simulink model "time_headway"  (R2019b)
settings: Solver=VariableStepAuto  StartTime=0.0  StopTime=10.0  RelTol=1e-3
libraries: robotlib x4
settings Model: Creator=ivory  LastModifiedBy=ivory

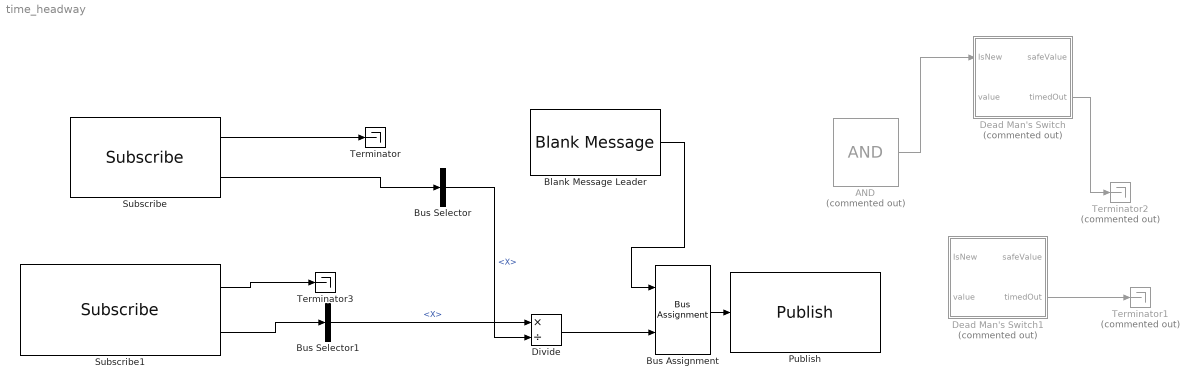
== system time_headway ==
  AND : Logic  Commented=on  IconShape=distinctive  AllPortsSameDT=off  OutDataTypeStr=boolean
  Blank Message Leader : robotlib/Blank Message  messageClass=Message  entityType=std_msgs/Float64  messageType=std_msgs/Float64  SampleTime=inf
      settings: SourceProductName=ROS Toolbox
  Bus Assignment : BusAssignment  AssignedSignals=Data
  Bus Selector : BusSelector  OutputSignals=Twist.Linear.X
  Bus Selector1 : BusSelector  OutputSignals=Point.X
  Dead Man's Switch : Subsystem  Commented=on  TreatAsAtomicUnit=on  mask{stepSize=0.05, timeout=0.2}
      mask prompts: stepSize "Simulation step size"; timeout "Timeout (in seconds)"
      mask help: Interprets whether a new message has been recently received, and if so permits the data in 'value' to be passed through. Otherwise, 0 is outputted from 'safeValue'
      mask Help: Interprets whether a new message has been recently received, and if so permits the data in 'value' to be passed through. Otherwise, 0 is outputted from 'safeValue'
  Dead Man's Switch1 : Subsystem  Commented=on  TreatAsAtomicUnit=on  mask{stepSize=0.05, timeout=0.2}
      mask prompts: stepSize "Simulation step size"; timeout "Timeout (in seconds)"
      mask help: Interprets whether a new message has been recently received, and if so permits the data in 'value' to be passed through. Otherwise, 0 is outputted from 'safeValue'
      mask Help: Interprets whether a new message has been recently received, and if so permits the data in 'value' to be passed through. Otherwise, 0 is outputted from 'safeValue'
  Divide : Product  Inputs=*/
  Publish : robotlib/Publish  topicSource=Select from ROS network  topic=/vehicle/timeheadway  messageType=geometry_msgs/Point  messageQueueLength=1
      settings: SourceProductName=ROS Toolbox
  Subscribe : robotlib/Subscribe  topicSource=Specify your own  topic=/vehicle/vel  messageType=geometry_msgs/TwistStamped  sampleTime=-1  messageQueueLength=1
      settings: SourceProductName=ROS Toolbox
  Subscribe1 : robotlib/Subscribe  topicSource=Specify your own  topic=/vehicle/distanceEstimator/dist  messageType=geometry_msgs/PointStamped  sampleTime=-1  messageQueueLength=1
      settings: SourceProductName=ROS Toolbox
  Terminator : Terminator
  Terminator1 : Terminator  Commented=on
  Terminator2 : Terminator  Commented=on
  Terminator3 : Terminator
  wires:
  Subscribe/1 -> Terminator/1
  Dead Man's Switch/2(timedOut) -> Terminator2/1
  Subscribe/2 -> Bus Selector/1
  Subscribe1/1 -> Terminator3/1
  AND/1 -> Dead Man's Switch/1(IsNew)
  Dead Man's Switch1/2(timedOut) -> Terminator1/1
  Subscribe1/2 -> Bus Selector1/1
  Bus Selector1/1 -> Divide/1  "<X>"
  Bus Selector/1 -> Divide/2  "<X>"
  Divide/1 -> Bus Assignment/2
  Blank Message Leader/1 -> Bus Assignment/1
  Bus Assignment/1 -> Publish/1

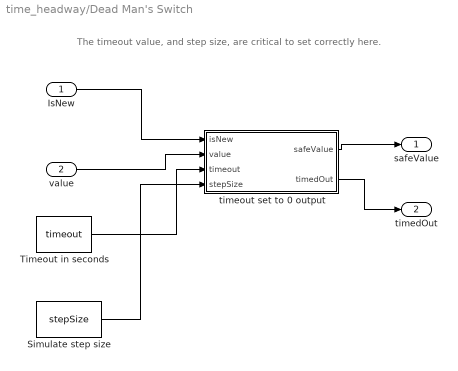
== system time_headway/Dead Man's Switch ==
  note: The timeout value, and step size, are critical to set correctly here.
  IsNew : Inport
  value : Inport  Port=2
  Simulate step size : Constant  Value=stepSize
  Timeout in seconds : Constant  Value=timeout
  timeout set to 0 output : MATLAB Function  TreatAsAtomicUnit=on
  safeValue : Outport  InitialOutput=[0]
  timedOut : Outport  Port=2  InitialOutput=[0]
  wires:
  IsNew/1 -> timeout set to 0 output/1(isNew)
  timeout set to 0 output/1(safeValue) -> safeValue/1
  value/1 -> timeout set to 0 output/2(value)
  Timeout in seconds/1 -> timeout set to 0 output/3(timeout)
  timeout set to 0 output/2(timedOut) -> timedOut/1
  Simulate step size/1 -> timeout set to 0 output/4(stepSize)

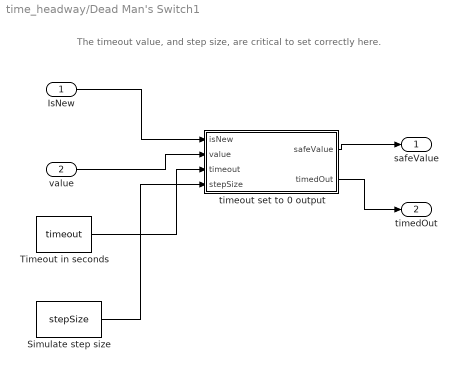
== system time_headway/Dead Man's Switch1 ==
  note: The timeout value, and step size, are critical to set correctly here.
  IsNew : Inport
  value : Inport  Port=2
  Simulate step size : Constant  Value=stepSize
  Timeout in seconds : Constant  Value=timeout
  timeout set to 0 output : MATLAB Function  TreatAsAtomicUnit=on
  safeValue : Outport  InitialOutput=[0]
  timedOut : Outport  Port=2  InitialOutput=[0]
  wires:
  Simulate step size/1 -> timeout set to 0 output/4(stepSize)
  timeout set to 0 output/2(timedOut) -> timedOut/1
  Timeout in seconds/1 -> timeout set to 0 output/3(timeout)
  value/1 -> timeout set to 0 output/2(value)
  timeout set to 0 output/1(safeValue) -> safeValue/1
  IsNew/1 -> timeout set to 0 output/1(isNew)

== matlab function time_headway/Dead Man's Switch1/timeout set to 0 output ==
  data: isNew input; safeValue output; value input; timeout input; timedOut output; stepSize input
function [safeValue,timedOut] = fcn(isNew,value,timeout,stepSize)
%#codegen
persistent sinceLastMsg
timedOut=true;
if isempty(sinceLastMsg)
    sinceLastMsg=(timeout/stepSize)+1;
end

safeValue=0;
% if no new message
% after timeout, we output 0
if( isNew == true )
    sinceLastMsg = 0;
else
    sinceLastMsg = sinceLastMsg+1;
end

% Note: we require step size as an input here, and depend on our
% system being executed at a regular rate, or bad things will happen
if( sinceLastMsg < timeout/stepSize )
    timedOut = false;
end
    
if( timedOut == false )
    safeValue = value;
end

== matlab function time_headway/Dead Man's Switch/timeout set to 0 output ==
  data: isNew input; safeValue output; value input; timeout input; timedOut output; stepSize input
function [safeValue,timedOut] = fcn(isNew,value,timeout,stepSize)
%#codegen
persistent sinceLastMsg
timedOut=true;
if isempty(sinceLastMsg)
    sinceLastMsg=(timeout/stepSize)+1;
end

safeValue=0;
% if no new message
% after timeout, we output 0
if( isNew == true )
    sinceLastMsg = 0;
else
    sinceLastMsg = sinceLastMsg+1;
end

% Note: we require step size as an input here, and depend on our
% system being executed at a regular rate, or bad things will happen
if( sinceLastMsg < timeout/stepSize )
    timedOut = false;
end
    
if( timedOut == false )
    safeValue = value;
end
